simulink library "tta"  (Simulink 8.1)
settings: Solver=ode1  StartTime=0.0  StopTime=Inf  FixedStep=0.001  RelTol=1e-3
PostLoadFcn:
  | , if any(exist('dsrtsu_mdlpostloadfcn', 'file') == [2, 3, 6]), try dsrtsu_mdlpostloadfcn('Execute', bdroot); catch fprintf('Error in PostLoadFcn (dsrtsu_mdlpostloadfcn) for model "%s":\n %s\n', bdroot, lasterr); end, end,
undefined symbols (not defined in the file or in its folder): KIFO_TTCDefault_s
libraries: hcu_lib x1
settings Model: DSRTSU_INTERNAL_RTI_VER=450  DSRTSU_INTERNAL_RTI_TYPE=rti1401  RTICANMMDATA=struct('GeneralSetupData',struct('modelroot','D:\ELN150201_TAIWAN\trunk\AdasDragon\software\sw_development\arch\app\ifo','generalsettings',struct('filesettings',struct('destfolder',struct('Name','RTICANMM_FILES','Check',1),'buildfolder',struct('Name','.','Check',1),'AbsDestfolder',struct('Name','D:\ELN150201_TAIWAN\trunk\AdasDragon\software\sw_development\arch\app\ifo\RTICANMM_FILES'),'AbsBuildfolder',struct('Name','D:\ELN150201_TAIWAN\trunk\AdasDragon\software\sw_development\arch\app\ifo'))),'options',struct('addpaths',1,'rmpaths',1,'addtrcexclusion',logical(1),'cannavigator',struct('checkmonitoring',0),'show_usrtrc',0,'use_usrtrc',0),'advanced',struct('options',[1 1 1 1 1 1 1 1 1 1 1 1 1 1 1 1 1 1 1 1 1 1 1 1 1 1 1 1 1 1 1 1 1 1 1 1 1 1 1 1 1 1 1 1 1 1 1 1 1 1 1 1 1 1 1 1 1 1 1 1 1 1 1 1 1 1 1 1 1 1 1 1 1 1 1 1 1 1 1 1 1 1 1 1 1 1 1 1 1 1 1 1 1 1 1 1 1 1 1 1]),'MPSetup',{{}},'modelname','tta','block','tta'))  DSRTSU_INTERNAL_RTIFPGA=40  Creator=AT015411  LastModifiedBy=AT015555

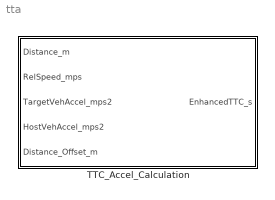
== system tta ==
  TTC_Accel_Calculation : Subsystem

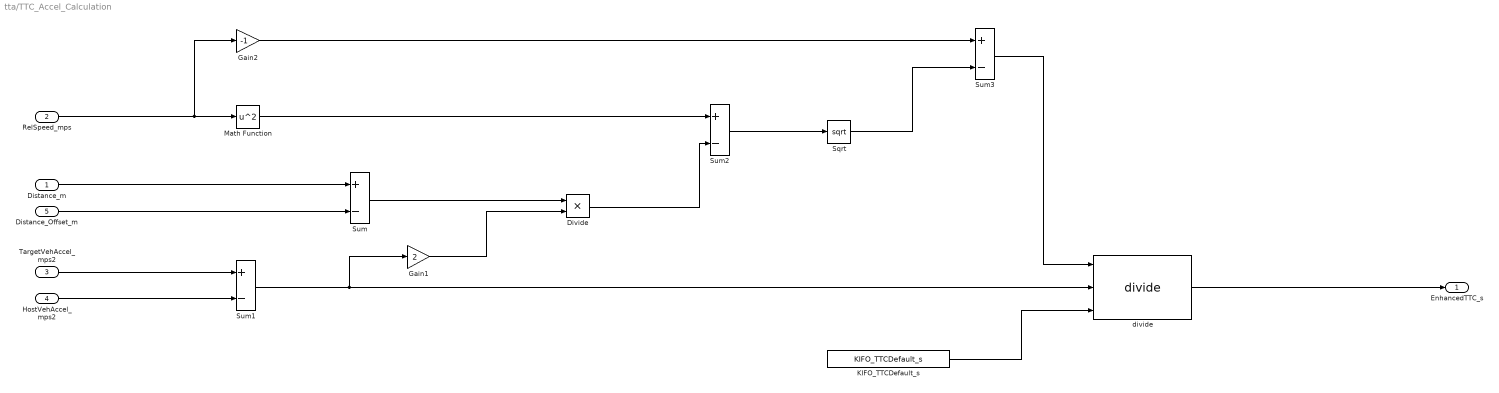
== system tta/TTC_Accel_Calculation ==
  Distance_m : Inport
  RelSpeed_mps : Inport  Port=2
  TargetVehAccel_mps2 : Inport  Port=3
  HostVehAccel_mps2 : Inport  Port=4
  Distance_Offset_m : Inport  Port=5
  Divide : Product  Inputs=**
  Gain1 : Gain  Gain=2
  Gain2 : Gain  Gain=-1
  KIFO_TTCDefault_s : Constant  Value=KIFO_TTCDefault_s
  Math Function : Math  Operator=square  SaturateOnIntegerOverflow=on
  Sqrt : Sqrt  SaturateOnIntegerOverflow=on
  Sum{,1..3} (4 alike) : Sum  Inputs=+-
  divide : hcu_lib/divide
  EnhancedTTC_s : Outport
  wires:
  Distance_m/1 -> Sum/1
  TargetVehAccel_mps2/1 -> Sum1/1
  HostVehAccel_mps2/1 -> Sum1/2
  Sum1/1 -> Gain1/1, divide/2
  RelSpeed_mps/1 -> Gain2/1, Math Function/1
  Sum/1 -> Divide/1
  Gain1/1 -> Divide/2
  Math Function/1 -> Sum2/1
  Divide/1 -> Sum2/2
  Sum2/1 -> Sqrt/1
  Gain2/1 -> Sum3/1
  Sqrt/1 -> Sum3/2
  Sum3/1 -> divide/1
  KIFO_TTCDefault_s/1 -> divide/3
  Distance_Offset_m/1 -> Sum/2
  divide/1 -> EnhancedTTC_s/1
